simulink model "SORU1_b-h"  (R2018b)
settings: Solver=VariableStepAuto  StartTime=0.0  StopTime=10.0  RelTol=1e-3
settings Model: Creator=Fatih  LastModifiedBy=Fatih

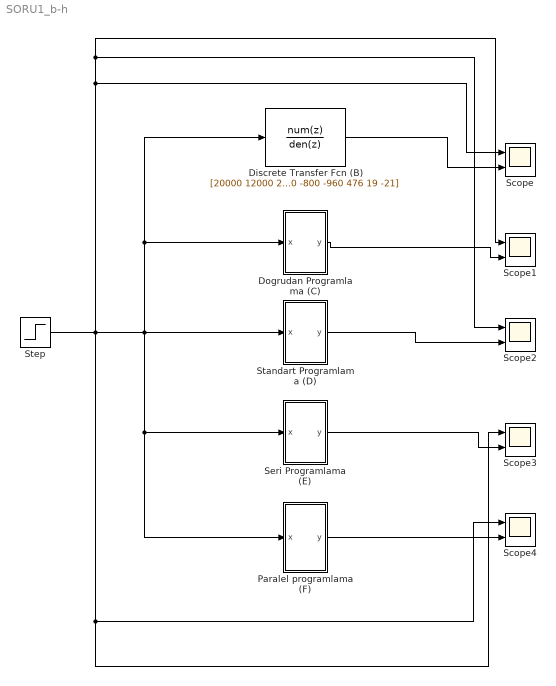
== system SORU1_b-h ==
  Discrete Transfer Fcn (B) : DiscreteTransferFcn  Numerator=[20000 12000 2800 3800 1450 0]  Denominator=[2000 -800 -960 476 19 -21]
  Dogrudan Programlama (C) : Subsystem
  Paralel programlama (F) : Subsystem
  Scope{,1..4} (5 alike) : Scope  NumInputPorts=2
  Seri Programlama (E) : Subsystem
  "Standart Programlama (D) " : Subsystem
  Step : Step  SampleTime=1
  wires:
  "Standart Programlama (D) "/1(y) -> Scope2/2
  Dogrudan Programlama (C)/1(y) -> Scope1/2
  Discrete Transfer Fcn (B)/1 -> Scope/2
  Seri Programlama (E)/1(y) -> Scope3/2
  Step/1 -> Scope4/1, Scope3/1, Scope1/1, Scope2/1, Scope/1, Paralel programlama (F)/1(x), Seri Programlama (E)/1(x), Dogrudan Programlama (C)/1(x), Discrete Transfer Fcn (B)/1, "Standart Programlama (D) "/1(x)
  Paralel programlama (F)/1(y) -> Scope4/2

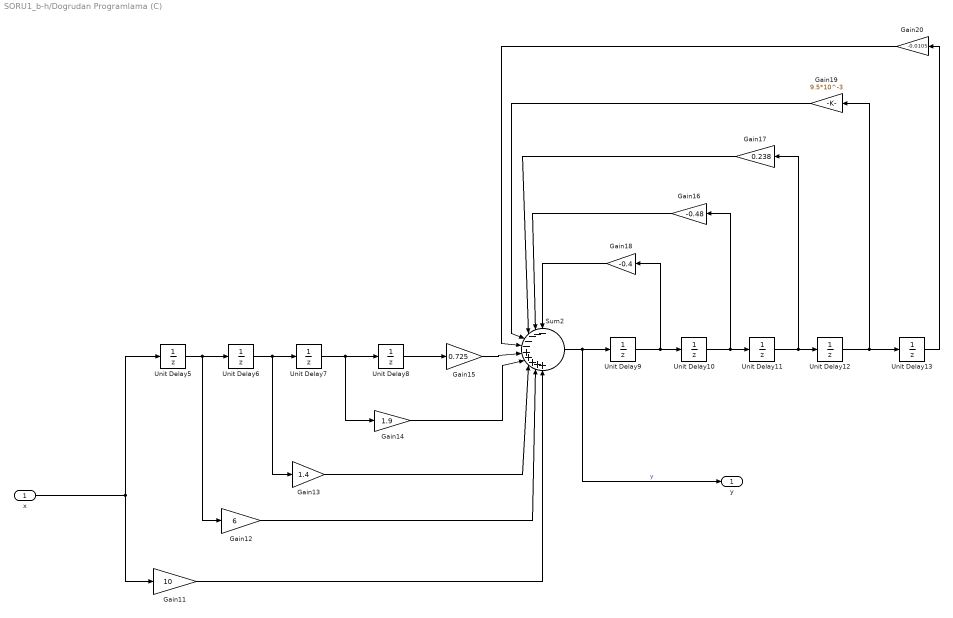
== system SORU1_b-h/Dogrudan Programlama (C) ==
  x : Inport
  Gain11 : Gain  Gain=10
  Gain12 : Gain  Gain=6
  Gain13 : Gain  Gain=1.4
  Gain14 : Gain  Gain=1.9
  Gain15 : Gain  Gain=0.725
  Gain16 : Gain  Gain=-0.48
  Gain17 : Gain  Gain=0.238
  Gain18 : Gain  Gain=-0.4
  Gain19 : Gain  Gain=9.5*10^-3
  Gain20 : Gain  Gain=-0.0105
  Sum2 : Sum  Inputs=-----+++++
  Unit Delay{5..13} (9 alike) : UnitDelay
  y : Outport
  wires:
  Gain13/1 -> Sum2/8
  Gain11/1 -> Sum2/10
  Gain18/1 -> Sum2/1
  Unit Delay13/1 -> Gain20/1
  Gain12/1 -> Sum2/9
  Gain17/1 -> Sum2/3
  Gain19/1 -> Sum2/4
  Unit Delay7/1 -> Gain14/1, Unit Delay8/1
  Unit Delay10/1 -> Gain16/1, Unit Delay11/1
  Gain15/1 -> Sum2/6
  Gain14/1 -> Sum2/7
  Unit Delay9/1 -> Gain18/1, Unit Delay10/1
  Unit Delay6/1 -> Gain13/1, Unit Delay7/1
  Unit Delay5/1 -> Gain12/1, Unit Delay6/1
  Unit Delay11/1 -> Gain17/1, Unit Delay12/1
  Unit Delay12/1 -> Unit Delay13/1, Gain19/1
  Gain16/1 -> Sum2/2
  Unit Delay8/1 -> Gain15/1
  x/1 -> Unit Delay5/1, Gain11/1
  Gain20/1 -> Sum2/5
  Sum2/1 -> y/1, Unit Delay9/1  "y"

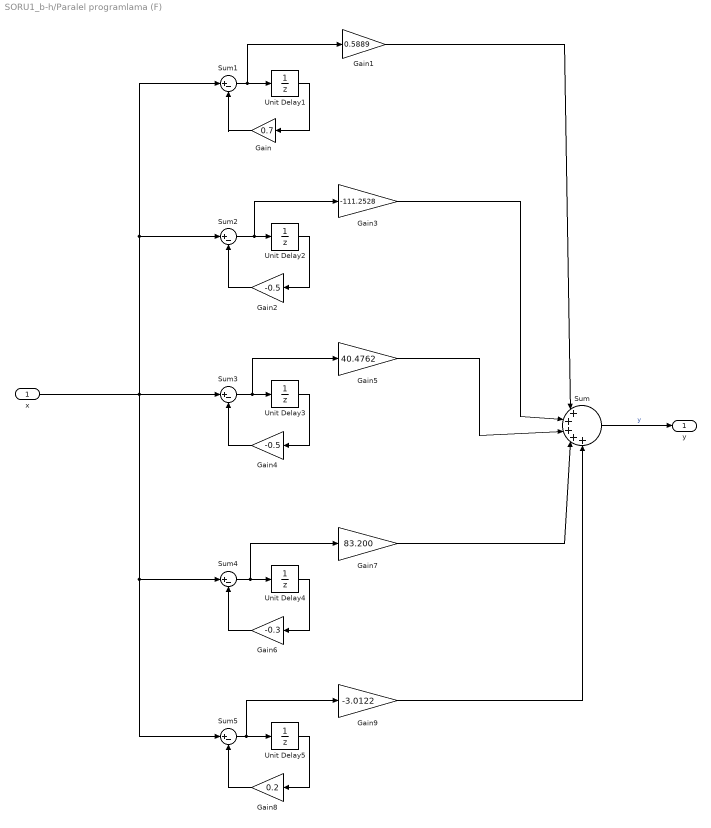
== system SORU1_b-h/Paralel programlama (F) ==
  x : Inport
  Gain : Gain  Gain=0.7
  Gain1 : Gain  Gain=0.5889
  Gain2 : Gain  Gain=-0.5
  Gain3 : Gain  Gain=-111.2528
  Gain4 : Gain  Gain=-0.5
  Gain5 : Gain  Gain=40.4762
  Gain6 : Gain  Gain=-0.3
  Gain7 : Gain  Gain=83.200
  Gain8 : Gain  Gain=0.2
  Gain9 : Gain  Gain=-3.0122
  Sum : Sum  Inputs=|+++++
  Sum{1..5} (5 alike) : Sum  Inputs=|+-
  Unit Delay{1..5} (5 alike) : UnitDelay
  y : Outport
  wires:
  Sum1/1 -> Gain1/1, Unit Delay1/1
  Gain8/1 -> Sum5/2
  Gain1/1 -> Sum/1
  Sum3/1 -> Gain5/1, Unit Delay3/1
  Gain5/1 -> Sum/3
  Unit Delay1/1 -> Gain/1
  Gain2/1 -> Sum2/2
  Gain3/1 -> Sum/2
  Gain4/1 -> Sum3/2
  Unit Delay4/1 -> Gain6/1
  Sum2/1 -> Gain3/1, Unit Delay2/1
  Gain6/1 -> Sum4/2
  Unit Delay2/1 -> Gain2/1
  Unit Delay3/1 -> Gain4/1
  Gain9/1 -> Sum/5
  Unit Delay5/1 -> Gain8/1
  Sum5/1 -> Gain9/1, Unit Delay5/1
  Sum4/1 -> Gain7/1, Unit Delay4/1
  Sum/1 -> y/1  "y"
  Gain/1 -> Sum1/2
  Gain7/1 -> Sum/4
  x/1 -> Sum5/1, Sum4/1, Sum3/1, Sum2/1, Sum1/1

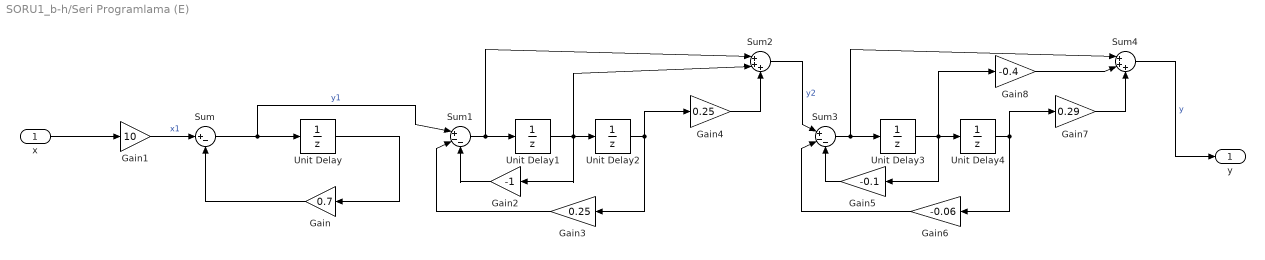
== system SORU1_b-h/Seri Programlama (E) ==
  x : Inport
  Gain : Gain  Gain=0.7
  Gain1 : Gain  Gain=10
  Gain2 : Gain  Gain=-1
  Gain3 : Gain  Gain=0.25
  Gain4 : Gain  Gain=0.25
  Gain5 : Gain  Gain=-0.1
  Gain6 : Gain  Gain=-0.06
  Gain7 : Gain  Gain=0.29
  Gain8 : Gain  Gain=-0.4
  Sum : Sum  Inputs=|+-
  Sum1 : Sum  Inputs=|+--
  Sum2 : Sum  Inputs=|+++
  Sum3 : Sum  Inputs=|+--
  Sum4 : Sum  Inputs=|+++
  Unit Delay{,1..4} (5 alike) : UnitDelay
  y : Outport
  wires:
  Sum4/1 -> y/1  "y"
  Gain1/1 -> Sum/1  "x1"
  Gain7/1 -> Sum4/3
  Gain4/1 -> Sum2/3
  Sum2/1 -> Sum3/1  "y2"
  Unit Delay4/1 -> Gain7/1, Gain6/1
  Gain8/1 -> Sum4/2
  Unit Delay1/1 -> Sum2/2, Gain2/1, Unit Delay2/1
  Unit Delay3/1 -> Gain8/1, Gain5/1, Unit Delay4/1
  Sum3/1 -> Sum4/1, Unit Delay3/1
  Sum1/1 -> Sum2/1, Unit Delay1/1
  Gain3/1 -> Sum1/2
  Unit Delay/1 -> Gain/1
  Gain/1 -> Sum/2
  Unit Delay2/1 -> Gain4/1, Gain3/1
  Gain5/1 -> Sum3/3
  Gain6/1 -> Sum3/2
  x/1 -> Gain1/1
  Gain2/1 -> Sum1/3
  Sum/1 -> Sum1/1, Unit Delay/1  "y1"

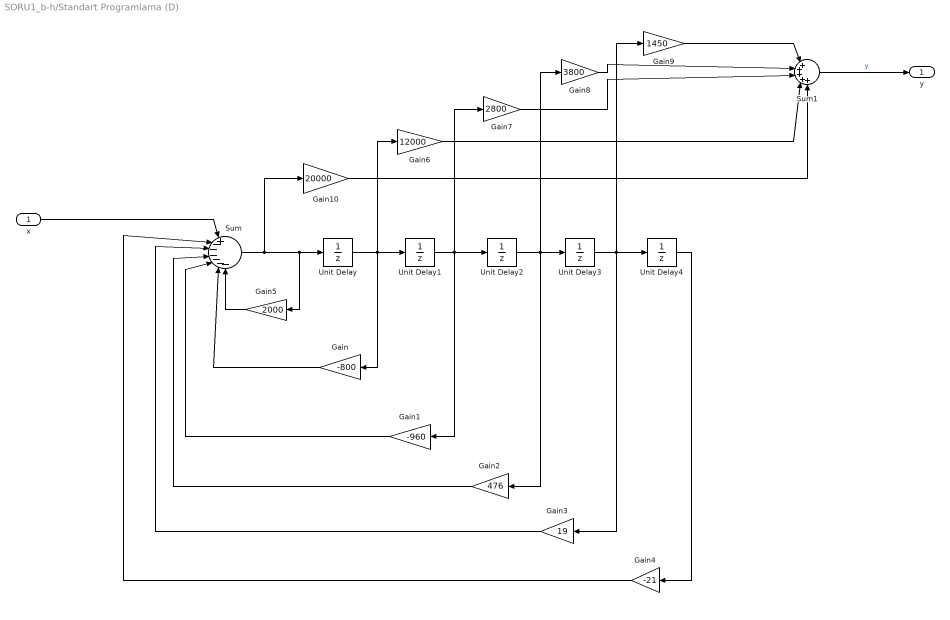
== system SORU1_b-h/Standart Programlama (D)  ==
  x : Inport
  Gain : Gain  Gain=-800
  Gain1 : Gain  Gain=-960
  Gain10 : Gain  Gain=20000
  Gain2 : Gain  Gain=476
  Gain3 : Gain  Gain=19
  Gain4 : Gain  Gain=-21
  Gain5 : Gain  Gain=2000
  Gain6 : Gain  Gain=12000
  Gain7 : Gain  Gain=2800
  Gain8 : Gain  Gain=3800
  Gain9 : Gain  Gain=1450
  Sum : Sum  Inputs=|+------
  Sum1 : Sum  Inputs=|+++++
  Unit Delay{,1..4} (5 alike) : UnitDelay
  y : Outport
  wires:
  Gain6/1 -> Sum1/4
  Gain10/1 -> Sum1/5
  Gain5/1 -> Sum/7
  Gain9/1 -> Sum1/1
  Unit Delay2/1 -> Gain8/1, Gain2/1, Unit Delay3/1
  x/1 -> Sum/1
  Gain8/1 -> Sum1/2
  Gain7/1 -> Sum1/3
  Unit Delay1/1 -> Gain7/1, Gain1/1, Unit Delay2/1
  Unit Delay3/1 -> Gain9/1, Gain3/1, Unit Delay4/1
  Sum1/1 -> y/1  "y"
  Gain3/1 -> Sum/3
  Gain2/1 -> Sum/4
  Gain1/1 -> Sum/5
  Gain/1 -> Sum/6
  Unit Delay/1 -> Gain6/1, Gain/1, Unit Delay1/1
  Gain4/1 -> Sum/2
  Unit Delay4/1 -> Gain4/1
  Sum/1 -> Gain10/1, Gain5/1, Unit Delay/1
